simulink model "Child"  (R2023a)
settings: Solver=FixedStepAuto  StartTime=0.0  StopTime=inf  RelTol=1e-3
libraries: androiduilib x6, androidsensorlib x3, androidaudiovideolib x3, androidcommunicationlib x3, fuzblock x1
settings Model: Creator=tamiz  LastModifiedBy=srira
settings OptimizationCC: EnhancedBackFolding=on  PassReuseOutputArgsAs=Individual arguments  ZeroExternalMemoryAtStartup=off  ZeroInternalMemoryAtStartup=off  MaxStackSize=64  OptimizeBlockOrder=speed  DifferentSizesBufferReuse=on  UseRowMajorAlgorithm=on  OptimizationCustomize=off  EfficientTunableParamExpr=on
settings DebuggingCC: ParameterTunabilityLossMsg=error
settings HardwareCC: ProdBitPerPointer=32  ProdBitPerSizeT=32  ProdBitPerPtrDiffT=32  ProdLargestAtomicInteger=Long  ProdLargestAtomicFloat=Double  ProdWordSize=32  ProdHWDeviceType=ARM Compatible->ARM Cortex  UseEmbeddedCoderFeatures=off  UseSimulinkCoderFeatures=off
settings RTWCC: Description=Embedded Coder  SystemTargetFile=ert.tlc  HardwareBoard=Android Device  TLCOptions="-aInlineSetEventsForThisBaseRateFcn=TLC_FALSE -aSuppressMultiTaskScheduler=TLC_FALSE  -aRateBasedStepFcn=0"  TemplateMakefile=ert_default_tmf  RTWVerbose=off  Toolchain=Android SDK/NDK Tools
settings CodeAppCC: ForceParamTrailComments=on  IgnoreCustomStorageClasses=off  OperatorAnnotations=on  SimulinkDataObjDesc=on  SFDataObjDesc=on  InsertBlockDesc=on
settings ERTTargetCC: SupportNonInlinedSFcns=on

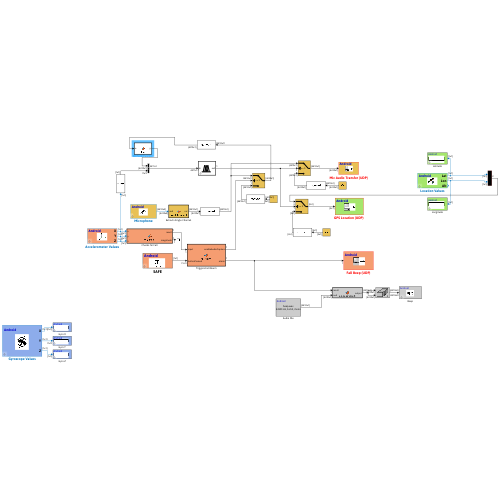
[thumbnail: Simulink's stored preview of the top-level diagram]
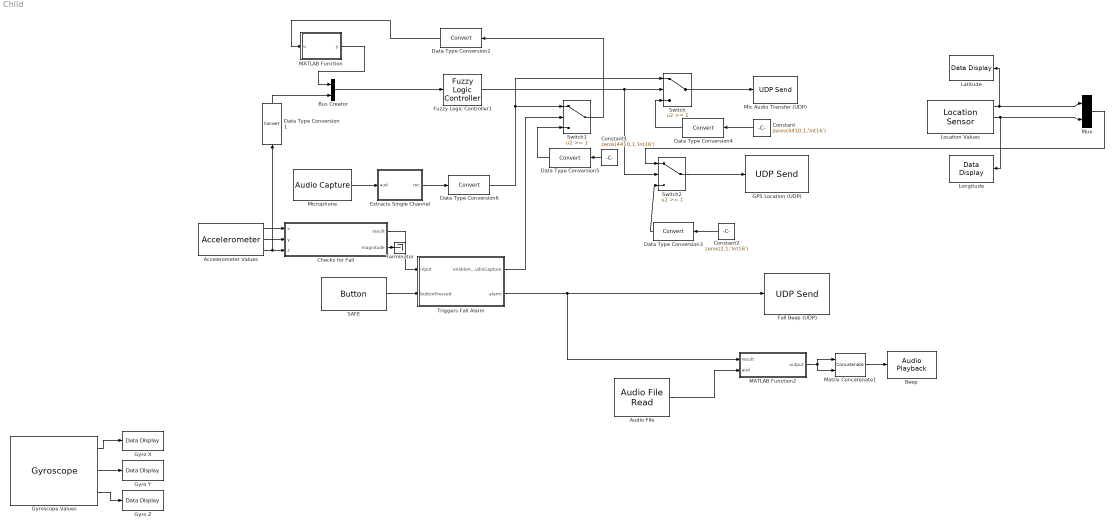
== system Child ==
  " SAFE " : androiduilib/Button  ButtonState=Not pressed  ButtonId=Child/_SAFE_  State=off  SampleTime=0.1  BlockPlatform=Android
  Accelerometer Values : androidsensorlib/Accelerometer  OutputVector=off  SampleTime=0.1  BlockPlatform=Android
  Audio FIle : androidaudiovideolib/Audio File Read  FileName=E:\IITGN\Child_Safety\beep.wav  FrameSize=4410
  Beep : androidaudiovideolib/Audio Playback  SampleFreq=44100  AudioSamplingFreq=44100  SampleTime=0.1  DeviceStr=0  QueueDuration=0  BlockPlatform=Android
  Bus Creator : BusCreator  Inputs=2
  Checks for Fall : MATLAB Function  TreatAsAtomicUnit=on
  Constant : Constant  Value=zeros(4410,1,'int16')  VectorParams1D=off
  Constant1 : Constant  Value=zeros(4410,1,'int16')  VectorParams1D=off
  Constant2 : Constant  Value=zeros(2,1,'int16')  VectorParams1D=off  OutDataTypeStr=Inherit: Inherit via back propagation
  Data Type Conversion{1..6} (6 alike) : DataTypeConversion  SaturateOnIntegerOverflow=off  RndMeth=Floor
  Extracts Single Channel : MATLAB Function  TreatAsAtomicUnit=on
  Fall Beep (UDP) : androidcommunicationlib/UDP Send  remoteURL='10.7.59.190'  remotePort=25001  localURL='0.0.0.0'  localPortSource=Automatically determine  localPort=-1  sampletime=-1  blockPlatform=Android  separateLengthPort=0
  Fuzzy Logic Controller1 : fuzblock/Fuzzy Logic  Controller  FIS='Control_Systems.fis'  OutputSampleNumber=101  DataType=double  FuzzifiedInputs=off  RuleFiringStrengths=off  RuleOutputs=off  AggregatedOutputs=off  SimulateUsing=Interpreted execution  OutOfRangeInputValueMessage=warning  NoRuleFiredMessage=warning  EmptyOutputFuzzySetMessage=warning
  "GPS Location (UDP) " : androidcommunicationlib/UDP Send  remoteURL='10.7.59.190'  remotePort=25000  localURL='0.0.0.0'  localPortSource=Automatically determine  localPort=-1  sampletime=-1  blockPlatform=Android  separateLengthPort=0
  Gyro X : androiduilib/Data Display  DataDisplayId=Child/Gyro_X  Format=Float  Precision=6  SimulateUsing=Code generation  blockPlatform=Android
  Gyro Y : androiduilib/Data Display  DataDisplayId=Child/Gyro_Y  Format=Float  Precision=6  SimulateUsing=Code generation  blockPlatform=Android
  Gyro Z : androiduilib/Data Display  DataDisplayId=Child/Gyro_Z  Format=Float  Precision=6  SimulateUsing=Code generation  blockPlatform=Android
  Gyroscope Values : androidsensorlib/Gyroscope  OutputVector=off  SampleTime=0.1  BlockPlatform=Android
  Latitude : androiduilib/Data Display  DataDisplayId=Child/Latitude  Format=Float  Precision=10  SimulateUsing=Code generation  blockPlatform=Android
  Location Values : androidsensorlib/Location Sensor  OutputVector=off  SampleTime=0.1  BlockPlatform=Android
  Longitude : androiduilib/Data Display  DataDisplayId=Child/Longitude  Format=Float  Precision=10  SimulateUsing=Code generation  blockPlatform=Android
  MATLAB Function : MATLAB Function  TreatAsAtomicUnit=on
  MATLAB Function2 : MATLAB Function  TreatAsAtomicUnit=on
  Matrix Concatenate1 : Concatenate  Mode=Multidimensional array  ConcatenateDimension=2
  Mic Audio Transfer (UDP) : androidcommunicationlib/UDP Send  remoteURL='10.7.59.190'  remotePort=25004  localURL='0.0.0.0'  localPortSource=Automatically determine  localPort=-1  sampletime=-1  blockPlatform=Android  separateLengthPort=0
  Microphone : androidaudiovideolib/Audio Capture  SampleFreq=44100  FrameSize=4410  SampleTime=0.1  SimulateUsing=Code generation  DeviceStr=0  QueueDuration=0  BlockPlatform=Android  AudioSamplingFreq=44100
  Mux : Mux  Inputs=2
  Switch : Switch  Threshold=1  SaturateOnIntegerOverflow=off  InputSameDT=off
  Switch1 : Switch  Threshold=1  SaturateOnIntegerOverflow=off  InputSameDT=off
  Switch2 : Switch  Threshold=1  OutDataTypeStr=Inherit: Inherit via back propagation  SaturateOnIntegerOverflow=off  InputSameDT=off
  Terminator : Terminator
  Triggers Fall Alarm : MATLAB Function  TreatAsAtomicUnit=on
  wires:
  Audio FIle/1 -> MATLAB Function2/2(aud)
  Location Values/1 -> Mux/1, Latitude/1
  Location Values/2 -> Longitude/1, Mux/2
  Accelerometer Values/1 -> Checks for Fall/1(x)
  Accelerometer Values/2 -> Checks for Fall/2(y)
  Accelerometer Values/3 -> Checks for Fall/3(z), Data Type Conversion1/1
  Gyroscope Values/1 -> Gyro X/1
  Gyroscope Values/2 -> Gyro Y/1
  Gyroscope Values/3 -> Gyro Z/1
  Matrix Concatenate1/1 -> Beep/1
  MATLAB Function2/1(output) -> Matrix Concatenate1/2, Matrix Concatenate1/1
  Triggers Fall Alarm/2(alarm) -> Fall Beep (UDP)/1, MATLAB Function2/1(result)
  " SAFE "/1 -> Triggers Fall Alarm/2(buttonPressed)
  Switch/1 -> Mic Audio Transfer (UDP)/1
  Constant/1 -> Data Type Conversion4/1
  Microphone/1 -> Extracts Single Channel/1(aud)
  Extracts Single Channel/1(rec) -> Data Type Conversion6/1
  Fuzzy Logic Controller1/1 -> Switch2/2, Switch/2
  Data Type Conversion1/1 -> Bus Creator/2
  Constant1/1 -> Data Type Conversion5/1
  Triggers Fall Alarm/1(enableAudioCapture) -> Switch1/2
  Switch1/1 -> Data Type Conversion2/1
  Constant2/1 -> Data Type Conversion3/1
  Switch2/1 -> "GPS Location (UDP) "/1
  Mux/1 -> Switch2/1
  Checks for Fall/2(magnitude) -> Terminator/1
  Checks for Fall/1(result) -> Triggers Fall Alarm/1(input)
  Data Type Conversion3/1 -> Switch2/3
  Data Type Conversion4/1 -> Switch/3
  Data Type Conversion5/1 -> Switch1/3
  Data Type Conversion6/1 -> Switch1/1, Switch/1
  Bus Creator/1 -> Fuzzy Logic Controller1/1
  Data Type Conversion2/1 -> MATLAB Function/1(u)
  MATLAB Function/1(y) -> Bus Creator/1

== matlab function Child/Checks for Fall ==
  data: x input; result output; y input; z input; magnitude output
function [result, magnitude] = checkFall(x, y, z)
    % Calculate the magnitude of acceleration
    magnitude = sqrt(x^2 + y^2 + z^2);
    acceleration_break_point = 60;
    % Check if magnitude is greater than or equal to 15
    if magnitude >= acceleration_break_point
        result = true;
    else
        result = false;
    end
end

== matlab function Child/MATLAB Function ==
  data: u input; y output
function y = fcn(u)
    y = mean(u(:));

== matlab function Child/MATLAB Function2 ==
  data: result input; output output; aud input
function output = processResult(result, aud)
    if result == 1
        output = aud;
    else
        output = zeros(4410,1,'int16');
    end
end

== matlab function Child/Triggers Fall Alarm ==
  data: enableAudioCapture output; input input; alarm output; buttonPressed input
function [enableAudioCapture, alarm] = fallAlarm(input, buttonPressed)
    persistent timerStarted;
    persistent danger;
    
    enableAudioCapture = 0;
    alarm = false;
    
    if isempty(danger)
        danger = 0;
    end

    if input == 1
        danger = 1;
        if isempty(timerStarted)
            timerStarted = true; 
            tic; % Start the timer
        end

        if timerStarted == false
            timerStarted = true; 
            tic; % Start the timer
        end
    end

    if danger == 1
        alarm = true;
        if toc >= 5 && buttonPressed ~= 1
            enableAudioCapture = 1;
        elseif buttonPressed == 1
            timerStarted = false;
            danger = 0;
            alarm = false; 
        end
    end
end

== matlab function Child/Extracts Single Channel ==
  data: aud input; rec output
function rec = singleChannel(aud)
    rec = aud(:,2);
